simulink model "OLTC_simulation"  (R2024a)
settings: Solver=ode45  StartTime=0.0  StopTime=0.1  RelTol=1e-3  EnableMultiTasking=on
libraries: spsIdealSwitchLib x8, spsRMSLib x4, spsCurrentMeasurementLib x3, spsSeriesRLCBranchLib x3, spsVoltageMeasurementLib x2, spsACVoltageSourceLib x1, spsMultiWindingTransformerLib x1, spspowerguiLib x1
settings Model: Creator=穷合  LastModifiedBy=49399
settings SolverCC: AlgebraicLoopSolver=TrustRegion
settings DataIOCC: ReturnWorkspaceOutputs=off
settings OptimizationCC: LifeSpan=inf
settings DebuggingCC: UnconnectedInputMsg=warning  UnconnectedOutputMsg=warning  UnconnectedLineMsg=warning  SFUnexpectedBacktrackingDiag=warning  SFNoUnconditionalDefaultTransitionDiag=warning  SFExecutionAtInitializationDiag=none  ArithmeticOperatorsInVariantConditions=warning
settings HardwareCC: ProdBitPerSizeT=32  ProdBitPerPtrDiffT=32  ProdWordSize=32  ProdHWDeviceType=Specified
settings SFSimCC: SimUseLocalCustomCode=off  CustomCodeUndefinedFunction=UseInterfaceOnly
settings RTWCC: RTWUseLocalCustomCode=off  GPUComputeCapability=3.5
settings CodeAppCC: StateflowObjectComments=on
settings GRTTargetCC: TargetLangStandard=C89/C90 (ANSI)
settings ConfigComp: CovMetricSettings=dw  CovSaveCumulativeToWorkspaceVar=on  CovSaveSingleToWorkspaceVar=on  CovExternalEMLEnable=off
settings SimscapeCC: SimscapeNormalizeSystem=off

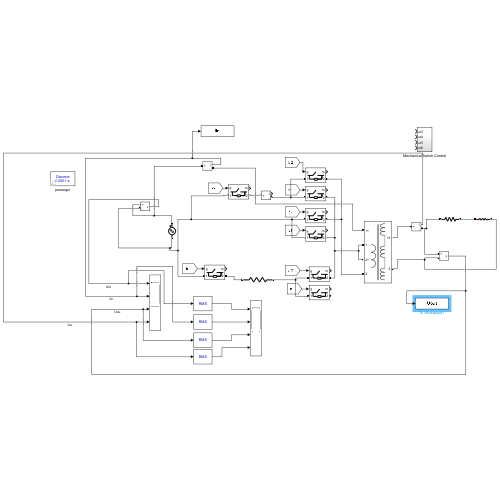
[thumbnail: Simulink's stored preview of the top-level diagram]
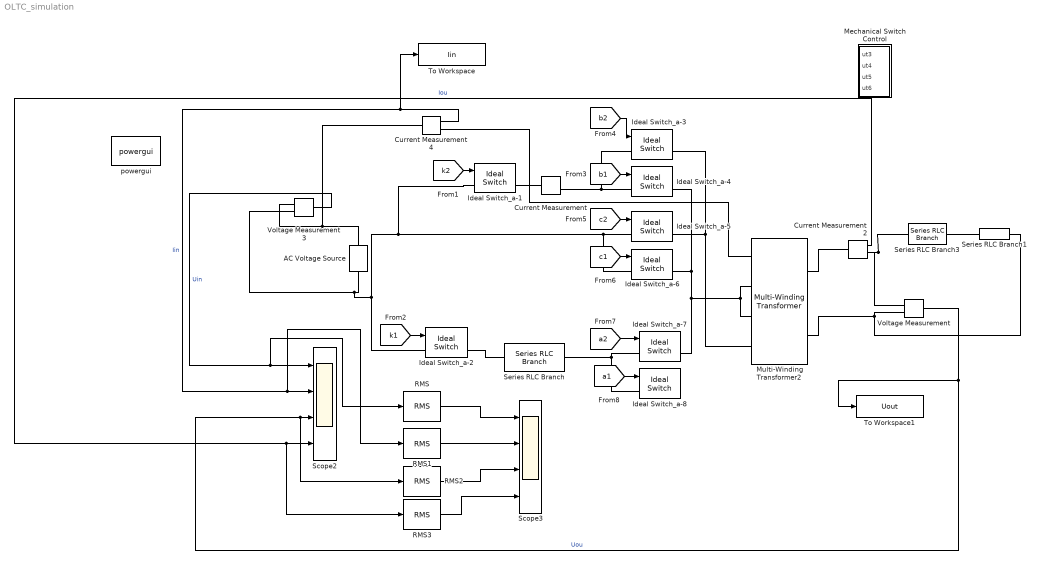
== system OLTC_simulation ==
  AC Voltage Source : spsACVoltageSourceLib/AC Voltage Source  Amplitude=5631.789  Phase=0  Frequency=50  SampleTime=0  Measurements=None  BusType=swing  Pref=10e3  Qref=0  Qmin=-inf  Qmax=+inf
  Current Measurement : spsCurrentMeasurementLib/Current Measurement  PhasorSimulation=off  OutputType=Complex  PSBequivalent=0
  Current Measurement2 : spsCurrentMeasurementLib/Current Measurement  PhasorSimulation=off  OutputType=Complex  PSBequivalent=0
  Current Measurement4 : spsCurrentMeasurementLib/Current Measurement  PhasorSimulation=off  OutputType=Complex  PSBequivalent=0
  Ideal Switch_a-{1..8} (8 alike) : spsIdealSwitchLib/Ideal Switch  Ron=0.0001  Lon=0  IC=0  Rs=1e10  Cs=inf  Measurements=on
  Mechanical Switch Control : Subsystem
  Multi-Winding Transformer2 : spsMultiWindingTransformerLib/Multi-Winding Transformer  LeftWindings=2  RightWindings=1  TappedWindings=no taps  NumberOfTaps=0  SetSaturation=off  Hysteresis=off  DataFile='hysteresis.mat'  Measurements=Winding voltages  UNITS=SI  NominalPower=[ 100e3 50]  NominalVoltages="[5773  577.3  230]"  WindingResistances="[0  0 0]"  WindingInductances=[0 0 0]  Rm=5000  Lm=5000  Saturation=[0 0;1.5085 48.617;628.54 61.582]  SpecifyInitialFlux=off  InitialFlux=0  BreakLoop=off  DiscreteSolver=Trapezoidal iterative  DataType=on  TransfoNumber=1
      settings: LibrarySourceBlock=|
      | sps_lib/Power Grid Elements/Multi-Winding
      | Transformer
  RMS{,1..3} (4 alike) : spsRMSLib/RMS  TrueRMS=on  Freq=50  RMSInit=120  Ts=0
  Scope2 : Scope  NumInputPorts=4
  Scope3 : Scope  NumInputPorts=4
  Series RLC Branch : spsSeriesRLCBranchLib/Series RLC Branch  LConnTagsString=__new0  RConnTagsString=__new0  BranchType=R  Resistance=3  Inductance=0  SetiL0=off  InitialCurrent=0  Capacitance=0  Setx0=off  InitialVoltage=0  Measurements=None
  Series RLC Branch1 : spsSeriesRLCBranchLib/Series RLC Branch  LConnTagsString=__new0  RConnTagsString=__new0  BranchType=R  Resistance=0.69256  Inductance=0  SetiL0=off  InitialCurrent=0  Capacitance=0  Setx0=off  InitialVoltage=0  Measurements=None
  Series RLC Branch3 : spsSeriesRLCBranchLib/Series RLC Branch  LConnTagsString=__new0  RConnTagsString=__new0  BranchType=R  Resistance=.1  Inductance=0  SetiL0=off  InitialCurrent=0  Capacitance=0  Setx0=off  InitialVoltage=0  Measurements=None
  To Workspace : ToWorkspace  VariableName=Iin  SaveFormat=Timeseries  SampleTime=-1
  To Workspace1 : ToWorkspace  VariableName=Uout  SaveFormat=Timeseries  SampleTime=-1
  Voltage Measurement : spsVoltageMeasurementLib/Voltage Measurement  PhasorSimulation=off  OutputType=Complex  PSBequivalent=0
  Voltage Measurement3 : spsVoltageMeasurementLib/Voltage Measurement  PhasorSimulation=off  OutputType=Complex  PSBequivalent=0
  powergui : spspowerguiLib/powergui  Priority=1  SimulationMode=Discrete  SampleTime=0.0001  frequency=60  Iterations=50  frequencyindice=50  Pbase=100e6  ErrMax=1e-4  UnitsV=kV  UnitsW=MW  buscounter=0  FunctionMessages=off  echomessages=off  EnableUseOfTLC=off  CurrentSourceSwitches=off  DisableSnubberDevices=off  DisableRonSwitches=off  DisableVfSwitches=off  DisplayEquations=off  AutomaticDiscreteSolvers=off  SolverType=Tustin/Backward Euler (TBE)  Interpol=off  ExternalGateDelay=off  methode=off  Ts=10  x0status=blocks  SPID=off  SwTol=0  HookPort=off  NonlinearTolerance=1e-4  nMaxIteration=100  ContinueOnMaxIteration=off  RestoreLinks=warning  ResistiveCurrentMeasurement=off  Frange=[0:2:500]  Ylog=off  Xlog=on  ShowGrid=off  save=off  variable=ZData  structure=0  ZoomFFT=off  StartTime=0.0  cycles=1  DisplayStyle=1  fundamental=60  FreqAxis=off  MaxFrequency=1000  frequencyindicesteady=1  RmsSteady=1  display=off
  wires:
  [k2] -> Ideal Switch_a-1/1
  [k1] -> Ideal Switch_a-2/1
  [b2] -> Ideal Switch_a-3/1
  [b1] -> Ideal Switch_a-4/1
  [c2] -> Ideal Switch_a-5/1
  [c1] -> Ideal Switch_a-6/1
  [a2] -> Ideal Switch_a-7/1
  [a1] -> Ideal Switch_a-8/1
  Voltage Measurement3/1 -> RMS/1, Scope2/1  "Uin"
  Current Measurement4/1 -> To Workspace/1, RMS1/1, Scope2/2  "Iin"
  Voltage Measurement/1 -> RMS2/1, Scope2/3, To Workspace1/1  "Uou"
  Current Measurement2/1 -> RMS3/1, Scope2/4  "Iou"
  RMS/1 -> Scope3/1
  RMS1/1 -> Scope3/2
  RMS2/1 -> Scope3/3
  RMS3/1 -> Scope3/4
  connections:
  Current Measurement/LConn1 -- Ideal Switch_a-1/RConn1
  Ideal Switch_a-2/RConn1 -- Series RLC Branch/LConn1
  Ideal Switch_a-7/LConn1 -- Ideal Switch_a-8/LConn1 -- Series RLC Branch/RConn1
  Ideal Switch_a-4/LConn1 -- Ideal Switch_a-3/LConn1 -- Current Measurement/RConn1
  Current Measurement2/RConn1 -- Series RLC Branch3/LConn1 -- Voltage Measurement/LConn1
  Multi-Winding Transformer2/RConn2 -- Series RLC Branch1/RConn1 -- Voltage Measurement/LConn2
  Ideal Switch_a-5/RConn1 -- Multi-Winding Transformer2/LConn4 -- Ideal Switch_a-3/RConn1
  Multi-Winding Transformer2/LConn2 -- Ideal Switch_a-7/RConn1 -- Ideal Switch_a-4/RConn1 -- Ideal Switch_a-6/RConn1 -- Multi-Winding Transformer2/LConn3
  Current Measurement2/LConn1 -- Multi-Winding Transformer2/RConn1
  Ideal Switch_a-1/LConn1 -- Ideal Switch_a-6/LConn1 -- Ideal Switch_a-5/LConn1 -- AC Voltage Source/LConn1 -- Voltage Measurement3/LConn2 -- Ideal Switch_a-2/LConn1
  Current Measurement4/RConn1 -- Multi-Winding Transformer2/LConn1
  Voltage Measurement3/LConn1 -- AC Voltage Source/RConn1 -- Current Measurement4/LConn1
  Series RLC Branch1/LConn1 -- Series RLC Branch3/RConn1

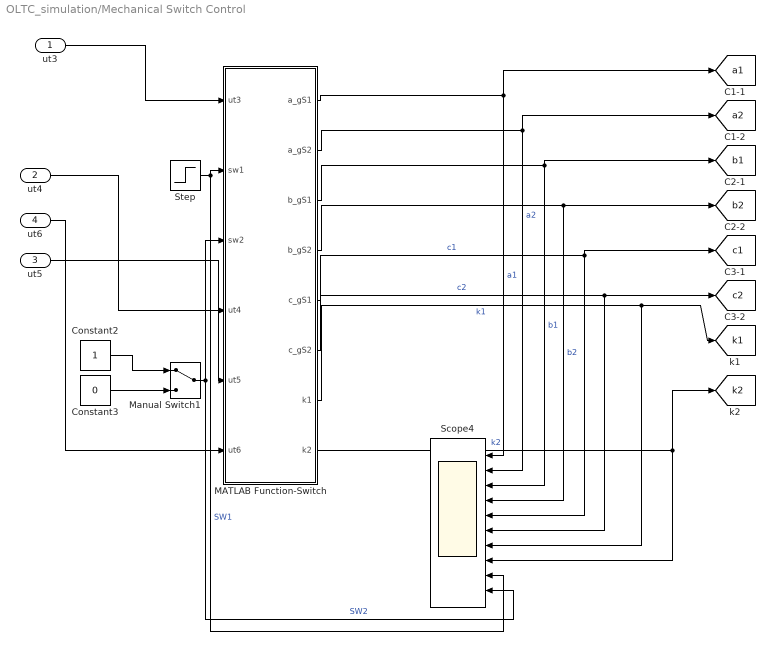
== system OLTC_simulation/Mechanical Switch Control ==
  ut3 : Inport
  ut4 : Inport  Port=2
  ut5 : Inport  Port=3
  ut6 : Inport  Port=4
  Constant2 : Constant
  Constant3 : Constant  Value=0
  MATLAB Function-Switch : MATLAB Function  TreatAsAtomicUnit=on
  Manual Switch1 : ManualSwitch
  Scope4 : Scope  NumInputPorts=10
  Step : Step  Time=5  SampleTime=0
  tag scope: a1=global, a2=global, b1=global, b2=global, c1=global, c2=global, k1=global, k2=global
  wires:
  MATLAB Function-Switch/1(a_gS1) -> [a1], Scope4/1  "a1"
  MATLAB Function-Switch/3(b_gS1) -> [b1], Scope4/3  "b1"
  MATLAB Function-Switch/6(c_gS2) -> [c2], Scope4/6  "c2"
  MATLAB Function-Switch/5(c_gS1) -> [c1], Scope4/5  "c1"
  MATLAB Function-Switch/4(b_gS2) -> [b2], Scope4/4  "b2"
  MATLAB Function-Switch/2(a_gS2) -> [a2], Scope4/2  "a2"
  MATLAB Function-Switch/7(k1) -> [k1], Scope4/7  "k1"
  MATLAB Function-Switch/8(k2) -> [k2], Scope4/8  "k2"
  Step/1 -> Scope4/9, MATLAB Function-Switch/2(sw1)  "SW1"
  Constant2/1 -> Manual Switch1/1
  Constant3/1 -> Manual Switch1/2
  Manual Switch1/1 -> Scope4/10, MATLAB Function-Switch/3(sw2)  "SW2"
  ut3/1 -> MATLAB Function-Switch/1(ut3)
  ut4/1 -> MATLAB Function-Switch/4(ut4)
  ut5/1 -> MATLAB Function-Switch/5(ut5)
  ut6/1 -> MATLAB Function-Switch/6(ut6)

== matlab function OLTC_simulation/Mechanical Switch Control/MATLAB Function-Switch ==
  data: ut3 input; a_gS1 output; a_gS2 output; b_gS1 output; b_gS2 output; sw1 input; c_gS1 output; c_gS2 output; k1 output; k2 output; sw2 input; ut4 input; ut5 input; ut6 input
function [a_gS1, a_gS2, b_gS1, b_gS2, c_gS1, c_gS2, k1, k2] = fcn(ut3, sw1, sw2, ut4, ut5, ut6)
%#codegen
% OLTC Control Logic Function - OLTC控制逻辑函数
% This function implements the control logic for an On-Load Tap Changer (OLTC)
% 此函数实现了有载分接开关(OLTC)的控制逻辑

% Declare persistent variables to maintain state between function calls
% 声明持久变量以在函数调用之间维持状态
persistent phase sw2pre num t1 ut1 ut2 ut7 a1 a2 b1 b2 c1 c2 k1t k2t;

% Initialize persistent variables if they are empty (first call)
% 如果持久变量为空(首次调用)，则初始化
if isempty(num)
   sw2pre = 0; phase = 0; num = 0;  % Initialize state tracking variables - 初始化状态跟踪变量
   t1 = 0;                          % Initial delay - 初始延迟
   
   % Timing parameters for switch operations (in milliseconds)
   % 开关操作的时间参数(单位：毫秒)
   ut1 = 90;  % Time for first operation (≥9ms) - 第一次操作的时间(≥9ms)
   ut2 = 80;  % Time for second operation (≥8ms) - 第二次操作的时间(≥8ms)
   % ut3, ut4, ut5, ut6 are passed as inputs to allow dynamic adjustment
   % ut3, ut4, ut5, ut6作为输入传递，允许动态调整
   ut7 = 100; % Time for final operation (≥10ms) - 最终操作的时间(≥10ms)
   
   % Initialize switch states (0=open, 1=closed)
   % 初始化开关状态(0=断开, 1=闭合)
   a1 = 0; a2 = 0;  % Main contacts A - A组主触点
   b1 = 0; b2 = 1;  % Main contacts B - B组主触点
   c1 = 0; c2 = 1;  % Auxiliary contacts C - C组辅助触点
   k1t = 0; k2t = 1; % Transition contacts K - K组过渡触点
end

% Assign output values from internal states
% 将内部状态分配给输出值
a_gS1 = a1; a_gS2 = a2;  % A group switch states - A组开关状态
b_gS1 = b1; b_gS2 = b2;  % B group switch states - B组开关状态
c_gS1 = c1; c_gS2 = c2;  % C group switch states - C组开关状态
k1 = k1t; k2 = k2t;      % K group switch states - K组开关状态

% Reset all states if main control switch is off
% 如果主控制开关关闭，则重置所有状态
if sw1 == 0
   sw2pre = 0; phase = 0; num = 0;
   t1 = 0;
   
   % Reset timing parameters
   % 重置时间参数
   ut1 = 90;  % ≥8ms
   ut2 = 80;  % ≥2.5ms
   ut7 = 100; % ≥10ms
   
   % Reset switch states to initial configuration
   % 将开关状态重置为初始配置
   a1 = 0; a2 = 0;
   b1 = 0; b2 = 1;
   c1 = 0; c2 = 1;
   k1t = 0; k2t = 1;
else
   % Increment counter if main switch is on
   % 如果主开关打开，则递增计数器
   num = num + 1;
end

% Detect rising and falling edges of control switch 2
% 检测控制开关2的上升沿和下降沿
if sw2 == 1 && sw2pre == 0
   num = 0; phase = 1; sw2pre = 1;  % Rising edge - Start tap up sequence - 上升沿-开始分接升压序列
elseif sw2 == 0 && sw2pre == 1
   num = 0; phase = 11; sw2pre = 0; % Falling edge - Start tap down sequence - 下降沿-开始分接降压序列
end

% State transition logic for tap up operation (phases 1-9)
% 分接升压操作的状态转换逻辑(阶段1-9)
if phase == 1 && num >= t1
   a2 = 1;                % Close contact A2 - 闭合触点A2
   phase = 2; num = 0;
elseif phase == 2 && num >= ut1
   c2 = 0; k1t = 1;       % Open C2, close K1 - 断开C2，闭合K1
   phase = 3; num = 0;
elseif phase == 3 && num >= ut2
   k2t = 0;               % Open K2 - 断开K2
   phase = 4; num = 0;
elseif phase == 4 && num >= ut3
   b2 = 0;                % Open B2 - 断开B2
   phase = 5; num = 0;
elseif phase == 5 && num >= ut4
   b1 = 1;                % Close B1 - 闭合B1
   phase = 6; num = 0;
elseif phase == 6 && num >= ut5
   k2t = 1;               % Close K2 - 闭合K2
   phase = 7; num = 0;
elseif phase == 7 && num >= ut6
   c1 = 1; k1t = 0;       % Close C1, open K1 - 闭合C1，断开K1
   phase = 8; num = 0;
elseif phase == 8 && num >= ut7
   a2 = 0;                % Open A2 - 断开A2
   phase = 9; num = 0;
elseif phase == 9 && num >= ut7
   num = 0;               % End of tap up sequence - 分接升压序列结束

% State transition logic for tap down operation (phases 11-19)
% 分接降压操作的状态转换逻辑(阶段11-19)
elseif phase == 11 && num >= t1
   a2 = 1;                % Close contact A2 - 闭合触点A2
   phase = 12; num = 0;
elseif phase == 12 && num >= ut1
   c1 = 0; k1t = 1;       % Open C1, close K1 - 断开C1，闭合K1
   phase = 13; num = 0;
elseif phase == 13 && num >= ut2
   k2t = 0;               % Open K2 - 断开K2
   phase = 14; num = 0;
elseif phase == 14 && num >= ut3
   b1 = 0;                % Open B1 - 断开B1
   phase = 15; num = 0;
elseif phase == 15 && num >= ut4
   b2 = 1;                % Close B2 - 闭合B2
   phase = 16; num = 0;
elseif phase == 16 && num >= ut5
   k2t = 1;               % Close K2 - 闭合K2
   phase = 17; num = 0;
elseif phase == 17 && num >= ut6
   c2 = 1; k1t = 0;       % Close C2, open K1 - 闭合C2，断开K1
   phase = 18; num = 0;
elseif phase == 18 && num >= ut7
   a2 = 0;                % Open A2 - 断开A2
   phase = 19; num = 0;
elseif phase == 19 && num >= ut7
   num = 0;               % End of tap down sequence - 分接降压序列结束
end
% End of state transition logic - 状态转换逻辑结束
end
